simulink model "lab3es1ver4"  (R2022a)
settings: Solver=VariableStepAuto  StartTime=0.0  StopTime=10.0  RelTol=1e-3
values from neighbouring files (symbols this model uses):
  g = 9.81    [VarLab3.m]
  Ie = I+m*l^2    (= 0.026047)    [VarLab3.m]
  l = 0.305    [VarLab3.m]
  m = 0.21    [VarLab3.m]
settings Model: Creator=bonvoltnuovo  LastModifiedBy=bonaventur
settings DebuggingCC: UnconnectedInputMsg=warning  UnconnectedOutputMsg=warning  UnconnectedLineMsg=warning
settings RTWCC: DLArmComputeVersion=19.05

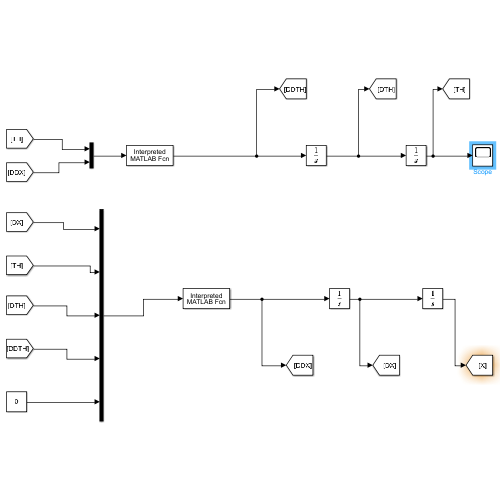
[thumbnail: Simulink's stored preview of the top-level diagram]
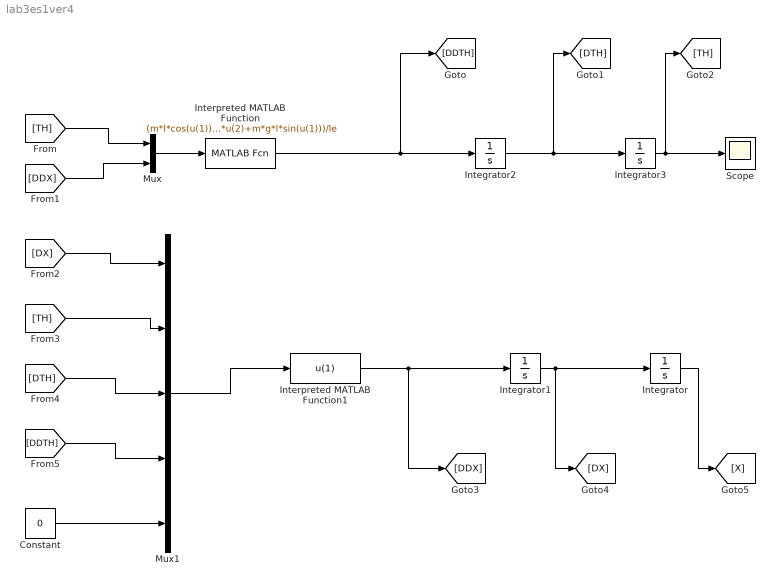
== system lab3es1ver4 ==
  Constant : Constant  Value=0
  Integrator : Integrator
  Integrator1 : Integrator
  Integrator2 : Integrator  InitialCondition=1
  Integrator3 : Integrator
  Interpreted MATLAB Function : MATLABFcn  MATLABFcn=(m*l*cos(u(1))*u(2)+m*g*l*sin(u(1)))/Ie
  Interpreted MATLAB Function1 : MATLABFcn  MATLABFcn=u(1)
  Mux : Mux  Inputs=2
  Mux1 : Mux  Inputs=5
  Scope : Scope
  wires:
  [DDX] -> Mux/2
  Mux/1 -> Interpreted MATLAB Function/1
  [TH] -> Mux/1
  Integrator2/1 -> Integrator3/1, [DTH]
  Integrator3/1 -> Scope/1, [TH]
  Interpreted MATLAB Function/1 -> [DDTH], Integrator2/1
  Constant/1 -> Mux1/5
  [DTH] -> Mux1/3
  [DX] -> Mux1/1
  [DDTH] -> Mux1/4
  Integrator1/1 -> Integrator/1, [DX]
  Integrator/1 -> [X]
  [TH] -> Mux1/2
  Mux1/1 -> Interpreted MATLAB Function1/1
  Interpreted MATLAB Function1/1 -> [DDX], Integrator1/1
